simulink model "questao_11"  (R2023a)
settings: Solver=VariableStepAuto  StartTime=0.0  StopTime=8*20  RelTol=1e-3
values from neighbouring files (symbols this model uses):
  A = pi*R^2    (= 16971.6689129)    [Aerogerador.m]
  b = 46e3    (= 46000)    [Aerogerador.m]
  Cpmax0 = Cpmax(:, 1)    [Aerogerador.m]
  Ea_nom = Pnom/ia_nom    [Aerogerador.m]
  ia_nom = x(2, :)    [Aerogerador.m]
  J = 9e6    (= 9000000)    [Aerogerador.m]
  kv = 900*2    (= 1800)    [Aerogerador.m]
  La = 108e-3    (= 0.108)    [Aerogerador.m]
  lambdaopt = 7.5    [Aerogerador.m]    (also in funNominal.m)
  R = 73.5    [Aerogerador.m]
  Ra = 100e-3    (= 0.1)    [Aerogerador.m]
  rho = 1.2    [Aerogerador.m]
  U_nom = x(1, :)    [Aerogerador.m]
  w_nom = (U_nom*lambdaopt)/R    [Aerogerador.m]
libraries: slpidlib x2, spsStairGeneratorLib x1
settings Model: Creator=danil  LastModifiedBy=danil

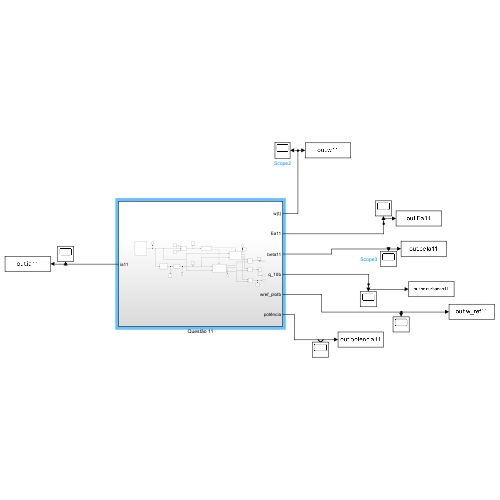
[thumbnail: Simulink's stored preview of the top-level diagram]
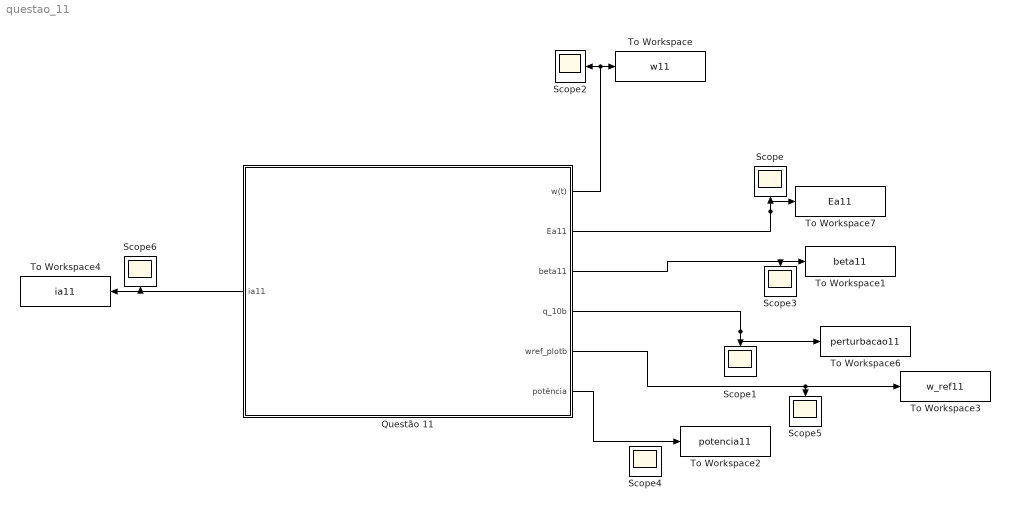
== system questao_11 ==
  Questão 11 : Subsystem
      settings: PortSchema="{\"entries\":[{\"content\":{\"sides\":[{\"content\":{\"connectorIds\":[\"Out7\"]},\"type\":\"ConnectorPlacement.EquallySpacedRectSide\",\"uuid\":\"401302fa-d1f5-4c54-ac19-93177bd2e6b7\"},{\"content\":{\"connectorIds\":[\"Out1\",\"Out2\",\"Out3\",\"Out4\",\"Out5\",\"Out6\"],\"side\":\"RIGHT\"},\"type\":\"ConnectorPlacement.EquallySpacedRectSide\",\"uuid\":\"3aac9436-5ff9-48c5-9773-0e70a06b410f\"},{\"content\":{\"side\":\"TOP\"},\"type\":\"ConnectorPlacement.EquallySpacedRectSide\",\"uuid\":\"07efa122-639e-46d6-af64-b4172f8f84f3\"}]},\"type\":\"ConnectorPlacement.EquallySpacedConnector\",\"uuid\":\"3685ca7e-51a8-437b-ae16-c8d6b387be2a\"}],\"packageUris\":[\"http://schema.mathworks.com/mf0/Connector/R2020b\"],\"version\":\"1.0\"}"
  Scope{,1..6} (7 alike) : Scope
  To Workspace : ToWorkspace  VariableName=w11  SampleTime=-1
      settings: Save2DSignal=2-D array (concatenate along first dimension)
  To Workspace1 : ToWorkspace  VariableName=beta11  SampleTime=-1
      settings: Save2DSignal=2-D array (concatenate along first dimension)
  To Workspace2 : ToWorkspace  VariableName=potencia11  SampleTime=-1
      settings: Save2DSignal=2-D array (concatenate along first dimension)
  To Workspace3 : ToWorkspace  VariableName=w_ref11  SampleTime=-1
      settings: Save2DSignal=2-D array (concatenate along first dimension)
  To Workspace4 : ToWorkspace  VariableName=ia11  SampleTime=-1
      settings: Save2DSignal=2-D array (concatenate along first dimension)
  To Workspace6 : ToWorkspace  VariableName=perturbacao11  SampleTime=-1
      settings: Save2DSignal=2-D array (concatenate along first dimension)
  To Workspace7 : ToWorkspace  VariableName=Ea11  SampleTime=-1
      settings: Save2DSignal=2-D array (concatenate along first dimension)
  wires:
  Questão 11/5(wref_plotb) -> To Workspace3/1, Scope5/1
  Questão 11/1(w(t)) -> To Workspace/1, Scope2/1
  Questão 11/4(q_10b) -> To Workspace6/1, Scope1/1
  Questão 11/2(Ea11) -> To Workspace7/1, Scope/1
  Questão 11/3(beta11) -> Scope3/1, To Workspace1/1
  Questão 11/6(potência) -> To Workspace2/1
  Questão 11/7(ia11) -> Scope6/1, To Workspace4/1

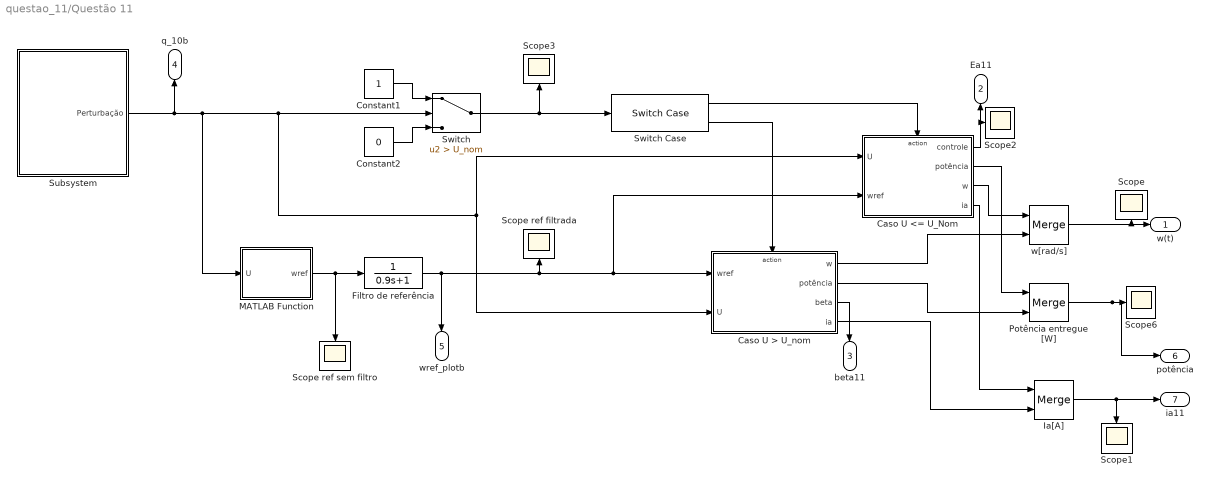
== system questao_11/Questão 11 ==
  Caso U <= U_Nom : Subsystem  TreatAsAtomicUnit=on
  Caso U > U_nom : Subsystem  TreatAsAtomicUnit=on
  Constant1 : Constant
  Constant2 : Constant  Value=0
  Filtro de referência : TransferFcn  Denominator=[0.9 1]
  Ia[A] : Merge
  MATLAB Function : MATLAB Function  TreatAsAtomicUnit=on
  Potência entregue [W] : Merge
  Scope{,1..3,6} (5 alike) : Scope
  Scope ref filtrada : Scope
  Scope ref sem filtro : Scope
  Subsystem : Subsystem
  Switch : Switch  Criteria=u2 > Threshold  Threshold=U_nom  SaturateOnIntegerOverflow=off  InputSameDT=off
  Switch Case : SwitchCase  CaseConditions={0, [1]}  ShowDefaultCase=off
  w[rad/s] : Merge
  w(t) : Outport
  Ea11 : Outport  Port=2
  beta11 : Outport  Port=3
  q_10b : Outport  Port=4
  wref_plotb : Outport  Port=5
  potência : Outport  Port=6
  ia11 : Outport  Port=7
  wires:
  Caso U <= U_Nom/3(w) -> w[rad/s]/1
  Switch/1 -> Scope3/1, Switch Case/1
  Switch Case/1 -> Caso U <= U_Nom/Action
  Constant2/1 -> Switch/3
  Switch Case/2 -> Caso U > U_nom/Action
  Caso U > U_nom/1(w) -> w[rad/s]/2
  Constant1/1 -> Switch/1
  Subsystem/1(Perturbação) -> Caso U > U_nom/2(U), Caso U <= U_Nom/1(U), Switch/2, MATLAB Function/1(U), q_10b/1
  w[rad/s]/1 -> Scope/1, w(t)/1
  Caso U <= U_Nom/1(controle) -> Scope2/1, Ea11/1
  MATLAB Function/1(wref) -> Filtro de referência/1, Scope ref sem filtro/1
  Caso U <= U_Nom/2(potência) -> Potência entregue [W]/1
  Caso U > U_nom/2(potência) -> Potência entregue [W]/2
  Potência entregue [W]/1 -> potência/1, Scope6/1
  Filtro de referência/1 -> Caso U <= U_Nom/2(wref), Caso U > U_nom/1(wref), Scope ref filtrada/1, wref_plotb/1
  Caso U > U_nom/3(beta) -> beta11/1
  Caso U > U_nom/4(ia) -> Ia[A]/2
  Ia[A]/1 -> Scope1/1, ia11/1
  Caso U <= U_Nom/4(ia) -> Ia[A]/1

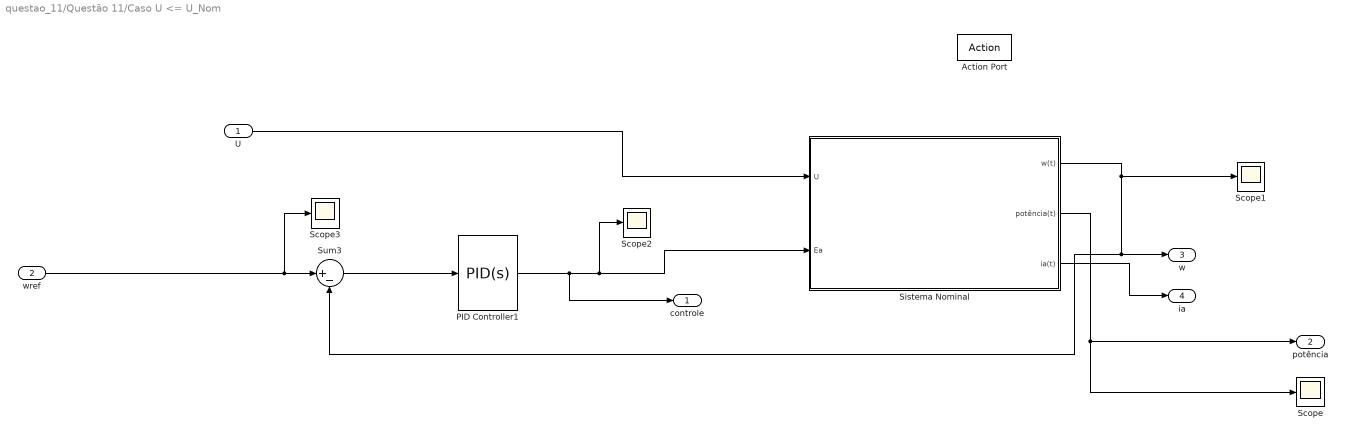
== system questao_11/Questão 11/Caso U <= U_Nom ==
  U : Inport
  wref : Inport  Port=2
  Action Port : ActionPort  ActionPortLabel=case [ 0 ]:
  PID Controller1 : slpidlib/PID Controller  Controller=PID  Form=Parallel  TimeDomain=Continuous-time  UseExternalTs=off  SampleTime=-1  IntegratorMethod=Forward Euler  FilterMethod=Forward Euler  ControllerParametersSource=internal  P=5586.71217162879  I=4755.74676167456  UseKiTs=off  D=1603.71676764274  N=478.091090181737  UseFilter=on  TunerSelectOption=Transfer Function Based (PID Tuner App)  InitialConditionSource=internal  InitialConditionForIntegrator=0  InitialConditionForFilter=0  DifferentiatorICPrevScaledInput=0  ExternalReset=none  TrackingMode=off  Kt=1  LimitOutput=on  SatLimitsSource=internal  UpperSaturationLimit=Ea_nom  LowerSaturationLimit=0  LinearizeAsGain=on  AntiWindupMode=none  Kb=1  LimitIntegrator=off  UpperIntegratorSaturationLimit=inf  LowerIntegratorSaturationLimit=-inf  POutMin=[]  POutMax=[]  IOutMin=[]  IOutMax=[]  DOutMin=[]  DOutMax=[]  NOutMin=[]  NOutMax=[]  SumOutMin=[]  SumOutMax=[]  SaturationOutMin=[]  SaturationOutMax=[]  PParamMin=[]  PParamMax=[]  IParamMin=[]  IParamMax=[]  DParamMin=[]  DParamMax=[]  NParamMin=[]  NParamMax=[]  KbParamMin=[]  KbParamMax=[]  KtParamMin=[]  KtParamMax=[]  KbOutMin=[]  KbOutMax=[]  KtOutMin=[]  KtOutMax=[]  IntegratorOutMin=[]  IntegratorOutMax=[]  FilterOutMin=[]  FilterOutMax=[]  SumI1OutMin=[]  SumI1OutMax=[]  SumI2OutMin=[]  SumI2OutMax=[]  SumI3OutMin=[]  SumI3OutMax=[]  SumI4OutMin=[]  SumI4OutMax=[]  SumDOutMin=[]  SumDOutMax=[]  DifferentiatorOutMin=[]  DifferentiatorOutMax=[]  FilterDiffOutCoefMin=[]  FilterDiffOutCoefMax=[]  ReciprocalOutMin=[]  ReciprocalOutMax=[]  SumDenOutMin=[]  SumDenOutMax=[]  SumNumOutMin=[]  SumNumOutMax=[]  DivideOutMin=[]  DivideOutMax=[]  UdiffTsProdOutMin=[]  UdiffTsProdOutMax=[]  NTsProdOutMin=[]  NTsProdOutMax=[]  UintegralTsProdOutMin=[]  UintegralTsProdOutMax=[]  UngainTsProdOutMin=[]  UngainTsProdOutMax=[]  ClampingZeroOutDataTypeStr=Inherit: Inherit via back propagation  ClampingZeroOutMin=[]  ClampingZeroOutMax=[]  FilterDenConstantOutDataTypeStr=Inherit: Inherit via back propagation  FilterDenConstantOutMin=[]  FilterDenConstantOutMax=[]  PCopyOutDataTypeStr=Inherit: Inherit via back propagation  PCopyOutMin=[]  PCopyOutMax=[]  NCopyOutDataTypeStr=Inherit: Inherit via back propagation  NCopyOutMin=[]  NCopyOutMax=[]  IntegratorContinuousStateAttributes=''  IntegratorStateMustResolveToSignalObject=off  IntegratorRTWStateStorageClass=Auto  FilterContinuousStateAttributes=''  FilterStateMustResolveToSignalObject=off  FilterRTWStateStorageClass=Auto  ParallelPVariant=InternalParameters  IdealPVariant=Disabled  IVariant=InternalParameters  DVariant=InternalParameters  IntegratorVariant=Continuous  SatVariant=Enabled  AWVariant=Passthrough  PCopyVariant=Disabled  TRVariant=Disabled  FdbkBlocksVariant=Forward  IdealPFdbkVariant=Disabled  SatFdbkVariant=Disabled  DerivativeFilterVariant=ContFilter  NVariant=InternalParameters  NCopyVariant=Disabled  FilterICVariant=InternalICsFilter  IntegratorICVariant=InternalICs  ExternalResetVariant=Disabled  TRSumVariant=Passthrough  SumFdbkVariant=Disabled  SumVariant=Sum_PID  TsampFilterVariant=InternalTs  TsampNgainVariant=Passthrough  TsampIntegralVariant=Disabled_SignalSpec  ExternalSaturationOutDataTypeStr=Inherit: Same as second input
  Scope{,1..3} (4 alike) : Scope
  Sistema Nominal : Subsystem
  Sum3 : Sum  Inputs=|+-
  controle : Outport
  potência : Outport  Port=2
  w : Outport  Port=3
  ia : Outport  Port=4
  wires:
  U/1 -> Sistema Nominal/1(U)
  Sistema Nominal/1(w(t)) -> w/1, Sum3/2, Scope1/1
  Sistema Nominal/2(potência(t)) -> Scope/1, potência/1
  PID Controller1/1 -> controle/1, Scope2/1, Sistema Nominal/2(Ea)
  Sum3/1 -> PID Controller1/1
  wref/1 -> Sum3/1, Scope3/1
  Sistema Nominal/3(ia(t)) -> ia/1

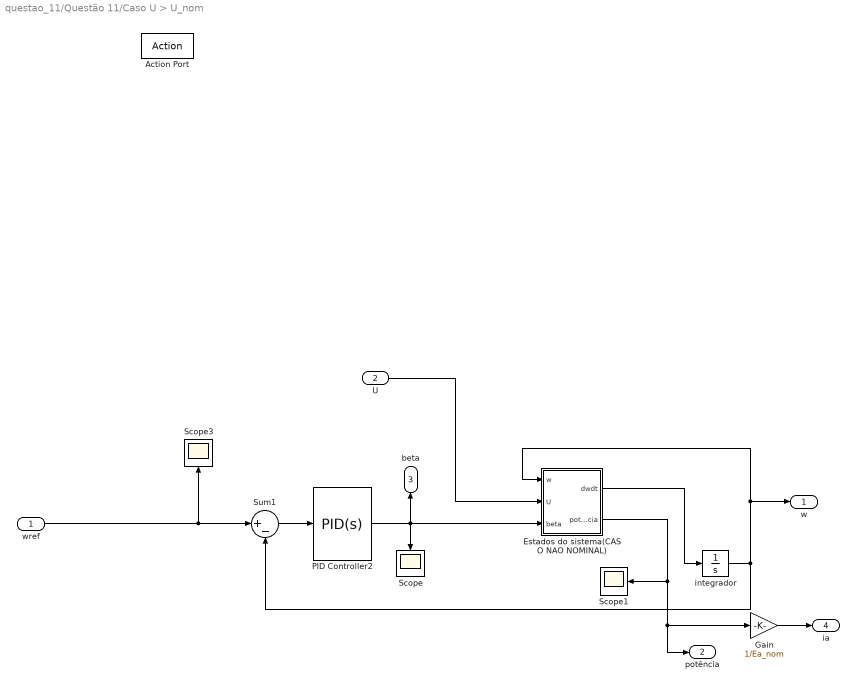
== system questao_11/Questão 11/Caso U > U_nom ==
  wref : Inport
  U : Inport  Port=2
  Action Port : ActionPort  ActionPortLabel=case [ 1 ]:
  Estados do sistema(CASO NAO NOMINAL) : MATLAB Function  TreatAsAtomicUnit=on
  Gain : Gain  Gain=1/Ea_nom
  PID Controller2 : slpidlib/PID Controller  Controller=PID  Form=Parallel  TimeDomain=Continuous-time  UseExternalTs=off  SampleTime=-1  IntegratorMethod=Forward Euler  FilterMethod=Forward Euler  ControllerParametersSource=internal  P=-0.410625599807359  I=-1.25025601800531  UseKiTs=off  D=0.00978955260280964  N=5.75949048000685  UseFilter=on  TunerSelectOption=Transfer Function Based (PID Tuner App)  InitialConditionSource=internal  InitialConditionForIntegrator=0  InitialConditionForFilter=0  DifferentiatorICPrevScaledInput=0  ExternalReset=none  TrackingMode=off  Kt=1  LimitOutput=off  SatLimitsSource=internal  UpperSaturationLimit=inf  LowerSaturationLimit=-inf  LinearizeAsGain=on  AntiWindupMode=none  Kb=1  LimitIntegrator=off  UpperIntegratorSaturationLimit=inf  LowerIntegratorSaturationLimit=-inf  POutMin=[]  POutMax=[]  IOutMin=[]  IOutMax=[]  DOutMin=[]  DOutMax=[]  NOutMin=[]  NOutMax=[]  SumOutMin=[]  SumOutMax=[]  SaturationOutMin=[]  SaturationOutMax=[]  PParamMin=[]  PParamMax=[]  IParamMin=[]  IParamMax=[]  DParamMin=[]  DParamMax=[]  NParamMin=[]  NParamMax=[]  KbParamMin=[]  KbParamMax=[]  KtParamMin=[]  KtParamMax=[]  KbOutMin=[]  KbOutMax=[]  KtOutMin=[]  KtOutMax=[]  IntegratorOutMin=[]  IntegratorOutMax=[]  FilterOutMin=[]  FilterOutMax=[]  SumI1OutMin=[]  SumI1OutMax=[]  SumI2OutMin=[]  SumI2OutMax=[]  SumI3OutMin=[]  SumI3OutMax=[]  SumI4OutMin=[]  SumI4OutMax=[]  SumDOutMin=[]  SumDOutMax=[]  DifferentiatorOutMin=[]  DifferentiatorOutMax=[]  FilterDiffOutCoefMin=[]  FilterDiffOutCoefMax=[]  ReciprocalOutMin=[]  ReciprocalOutMax=[]  SumDenOutMin=[]  SumDenOutMax=[]  SumNumOutMin=[]  SumNumOutMax=[]  DivideOutMin=[]  DivideOutMax=[]  UdiffTsProdOutMin=[]  UdiffTsProdOutMax=[]  NTsProdOutMin=[]  NTsProdOutMax=[]  UintegralTsProdOutMin=[]  UintegralTsProdOutMax=[]  UngainTsProdOutMin=[]  UngainTsProdOutMax=[]  ClampingZeroOutDataTypeStr=Inherit: Inherit via back propagation  ClampingZeroOutMin=[]  ClampingZeroOutMax=[]  FilterDenConstantOutDataTypeStr=Inherit: Inherit via back propagation  FilterDenConstantOutMin=[]  FilterDenConstantOutMax=[]  PCopyOutDataTypeStr=Inherit: Inherit via back propagation  PCopyOutMin=[]  PCopyOutMax=[]  NCopyOutDataTypeStr=Inherit: Inherit via back propagation  NCopyOutMin=[]  NCopyOutMax=[]  IntegratorContinuousStateAttributes=''  IntegratorStateMustResolveToSignalObject=off  IntegratorRTWStateStorageClass=Auto  FilterContinuousStateAttributes=''  FilterStateMustResolveToSignalObject=off  FilterRTWStateStorageClass=Auto  ParallelPVariant=InternalParameters  IdealPVariant=Disabled  IVariant=InternalParameters  DVariant=InternalParameters  IntegratorVariant=Continuous  SatVariant=Disabled  AWVariant=Passthrough  PCopyVariant=Disabled  TRVariant=Disabled  FdbkBlocksVariant=Forward  IdealPFdbkVariant=Disabled  SatFdbkVariant=Disabled  DerivativeFilterVariant=ContFilter  NVariant=InternalParameters  NCopyVariant=Disabled  FilterICVariant=InternalICsFilter  IntegratorICVariant=InternalICs  ExternalResetVariant=Disabled  TRSumVariant=Passthrough  SumFdbkVariant=Disabled  SumVariant=Sum_PID  TsampFilterVariant=InternalTs  TsampNgainVariant=Passthrough  TsampIntegralVariant=Disabled_SignalSpec  ExternalSaturationOutDataTypeStr=Inherit: Same as second input
  Scope : Scope
  Scope1 : Scope
  Scope3 : Scope
  Sum1 : Sum  Inputs=|+-
  integrador : Integrator  InitialCondition=w_nom
  w : Outport
  potência : Outport  Port=2
  beta : Outport  Port=3
  ia : Outport  Port=4
  wires:
  Estados do sistema(CASO NAO NOMINAL)/1(dwdt) -> integrador/1
  integrador/1 -> Sum1/2, Estados do sistema(CASO NAO NOMINAL)/1(w), w/1
  PID Controller2/1 -> Estados do sistema(CASO NAO NOMINAL)/3(beta), Scope/1, beta/1
  Sum1/1 -> PID Controller2/1
  U/1 -> Estados do sistema(CASO NAO NOMINAL)/2(U)
  Estados do sistema(CASO NAO NOMINAL)/2(potencia) -> Gain/1, potência/1, Scope1/1
  wref/1 -> Sum1/1, Scope3/1
  Gain/1 -> ia/1

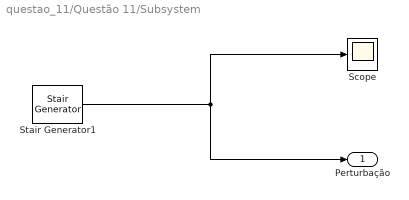
== system questao_11/Questão 11/Subsystem ==
  Scope : Scope
  Stair Generator1 : spsStairGeneratorLib/Stair Generator  t=vecstepinterval  e=vecU11  Ts=0
  Perturbação : Outport
  wires:
  Stair Generator1/1 -> Scope/1, Perturbação/1

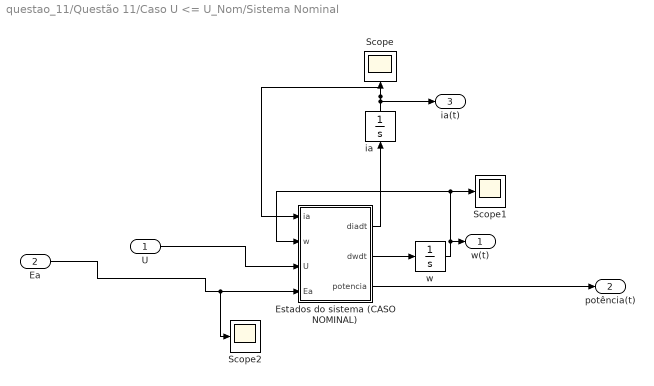
== system questao_11/Questão 11/Caso U <= U_Nom/Sistema Nominal ==
  U : Inport
  Ea : Inport  Port=2
  Estados do sistema (CASO NOMINAL) : MATLAB Function  TreatAsAtomicUnit=on
  Scope : Scope
  Scope1 : Scope
  Scope2 : Scope
  ia : Integrator  InitialCondition=1
  w : Integrator  InitialCondition=6.1e-2
  w(t) : Outport
  potência(t) : Outport  Port=2
  ia(t) : Outport  Port=3
  wires:
  Estados do sistema (CASO NOMINAL)/2(dwdt) -> w/1
  Estados do sistema (CASO NOMINAL)/1(diadt) -> ia/1
  ia/1 -> ia(t)/1, Estados do sistema (CASO NOMINAL)/1(ia), Scope/1
  Ea/1 -> Scope2/1, Estados do sistema (CASO NOMINAL)/4(Ea)
  U/1 -> Estados do sistema (CASO NOMINAL)/3(U)
  Estados do sistema (CASO NOMINAL)/3(potencia) -> potência(t)/1
  w/1 -> Scope1/1, Estados do sistema (CASO NOMINAL)/2(w), w(t)/1

== matlab function questao_11/Questão 11/MATLAB Function ==
  data: U input; wref output; R parameter; lambdaopt parameter
function wref = fcn(U, R, lambdaopt)

wref = (lambdaopt*U)/R;

== matlab function questao_11/Questão 11/Caso U <= U_Nom/Sistema Nominal/Estados do sistema (CASO NOMINAL) ==
  data: ia input; w input; diadt output; dwdt output; U input; Ra parameter; J parameter; Cpmax0 parameter; A parameter; b parameter; kv parameter; La parameter; rho parameter; Ea input; potencia output
function [diadt, dwdt, potencia] = fcn(ia, w, U, Ra, J, Cpmax0, A, b, kv, La, rho, Ea)



diadt = (1/La) * (kv*w - Ra*ia - Ea);
dwdt = (1/J) * ((Cpmax0*0.5*rho*A*U^3)/w - b*w - kv*ia);
potencia = Ea*ia;

== matlab function questao_11/Questão 11/Caso U > U_nom/Estados do sistema(CASO NAO NOMINAL) ==
  data: w input; dwdt output; U input; J parameter; A parameter; b parameter; kv parameter; rho parameter; ia_nom parameter; beta input; lambdaopt parameter; potencia output; Ea_nom parameter
function [dwdt, potencia]  = fcn(w, U, J, A, b, kv, rho, ia_nom, beta, lambdaopt, Ea_nom)


Cp = (0.44 - 0.167*beta)*sin((pi*lambdaopt)/(15 - 0.3*beta)) - 0.16*lambdaopt*beta;

dwdt = (1/J) * ((Cp*0.5*rho*A*U^3)/w - b*w - kv*ia_nom);

potencia = Ea_nom*ia_nom;
